simulink model "save"  (R2021a)
settings: Solver=ode4  StartTime=0.0  StopTime=100  FixedStep=0.01  MaxStep=0.01  RelTol=1e-4  EnableMultiTasking=on
undefined symbols (not defined in the file or in its folder): g, k1, k2, k3, m
libraries: pid_lib x1
settings Model: Creator=zlioo  LastModifiedBy=zlioo
settings SolverCC: AlgebraicLoopSolver=TrustRegion
settings DataIOCC: LimitDataPoints=on  SaveOutput=off  SaveTime=off
settings OptimizationCC: ExpressionDepthLimit=2147483647  LifeSpan=1
settings DebuggingCC: UnderspecifiedInitializationDetection=Classic  MergeDetectMultiDrivingBlocksExec=none  FcnCallInpInsideContextMsg=warning  AllowSymbolicDim=off  StateNameClashWarn=warning  SFUnexpectedBacktrackingDiag=warning  SFNoUnconditionalDefaultTransitionDiag=warning  SFExecutionAtInitializationDiag=none  SFMachineParentedDataDiag=warning  ArithmeticOperatorsInVariantConditions=warning
settings SFSimCC: SimUseLocalCustomCode=off  CustomCodeUndefinedFunction=UseInterfaceOnly
settings RTWCC: RTWUseLocalCustomCode=off
settings CodeAppCC: StateflowObjectComments=on
settings GRTTargetCC: TargetLangStandard=C89/C90 (ANSI)  CombineOutputUpdateFcns=off  GRTInterface=on

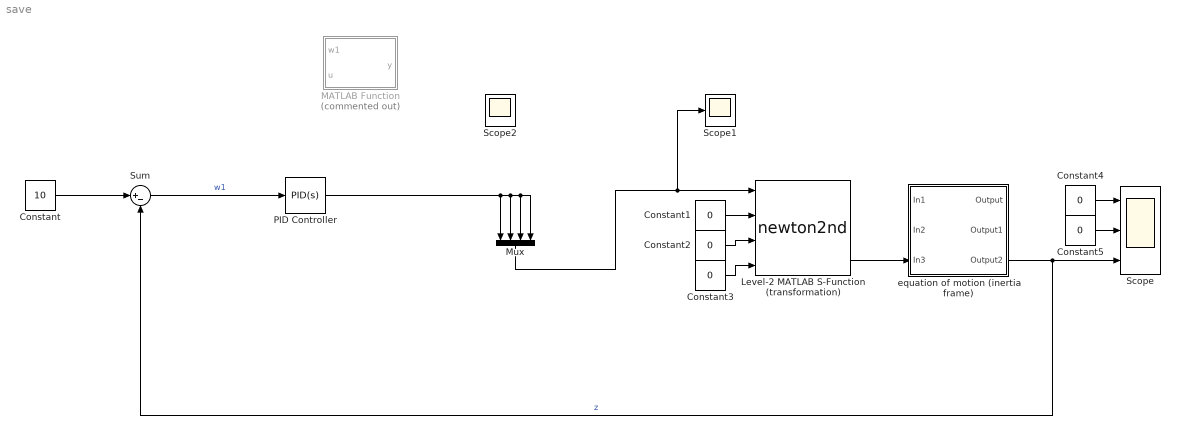
== system save ==
  Constant : Constant  Value=10
  Constant{1..5} (5 alike) : Constant  Value=0
  Level-2 MATLAB S-Function (transformation) : M-S-Function  FunctionName=newton2nd
  MATLAB Function : MATLAB Function  Commented=on  TreatAsAtomicUnit=on
  Mux : Mux
  PID Controller : pid_lib/PID Controller  Controller=PID  Form=Parallel  TimeDomain=Continuous-time  UseExternalTs=off  SampleTime=-1  IntegratorMethod=Forward Euler  FilterMethod=Forward Euler  ControllerParametersSource=internal  P=1.35772493107891  I=0.277456410616241  D=1.63144377299047  UseFilter=on  N=23.8074436453229  TunerSelectOption=Transfer Function Based (PID Tuner App)  InitialConditionSource=internal  InitialConditionForIntegrator=0  InitialConditionForFilter=0  DifferentiatorICPrevScaledInput=0  ExternalReset=none  TrackingMode=off  Kt=1  LimitOutput=off  SatLimitsSource=internal  UpperSaturationLimit=Inf  LowerSaturationLimit=0  LinearizeAsGain=on  AntiWindupMode=none  Kb=1  POutMin=[]  POutMax=[]  IOutMin=[]  IOutMax=[]  DOutMin=[]  DOutMax=[]  NOutMin=[]  NOutMax=[]  SumOutMin=[]  SumOutMax=[]  SaturationOutMin=[]  SaturationOutMax=[]  PParamMin=[]  PParamMax=[]  IParamMin=[]  IParamMax=[]  DParamMin=[]  DParamMax=[]  NParamMin=[]  NParamMax=[]  KbParamMin=[]  KbParamMax=[]  KtParamMin=[]  KtParamMax=[]  KbOutMin=[]  KbOutMax=[]  KtOutMin=[]  KtOutMax=[]  IntegratorOutMin=[]  IntegratorOutMax=[]  FilterOutMin=[]  FilterOutMax=[]  SumI1OutMin=[]  SumI1OutMax=[]  SumI2OutMin=[]  SumI2OutMax=[]  SumI3OutMin=[]  SumI3OutMax=[]  SumI4OutMin=[]  SumI4OutMax=[]  SumDOutMin=[]  SumDOutMax=[]  DifferentiatorOutMin=[]  DifferentiatorOutMax=[]  FilterDiffOutCoefMin=[]  FilterDiffOutCoefMax=[]  ReciprocalOutMin=[]  ReciprocalOutMax=[]  SumDenOutMin=[]  SumDenOutMax=[]  SumNumOutMin=[]  SumNumOutMax=[]  DivideOutMin=[]  DivideOutMax=[]  UdiffTsProdOutMin=[]  UdiffTsProdOutMax=[]  NTsProdOutMin=[]  NTsProdOutMax=[]  UintegralTsProdOutMin=[]  UintegralTsProdOutMax=[]  UngainTsProdOutMin=[]  UngainTsProdOutMax=[]  IntegratorContinuousStateAttributes=''  IntegratorStateMustResolveToSignalObject=off  IntegratorRTWStateStorageClass=Auto  FilterContinuousStateAttributes=''  FilterStateMustResolveToSignalObject=off  FilterRTWStateStorageClass=Auto  ParallelPVariant=InternalParameters  IdealPVariant=Disabled  IVariant=InternalParameters  DVariant=InternalParameters  IntegratorVariant=Continuous  SatVariant=Disabled  AWVariant=Passthrough  PCopyVariant=Disabled  TRVariant=Disabled  FdbkBlocksVariant=Forward  IdealPFdbkVariant=Disabled  SatFdbkVariant=Disabled  DerivativeFilterVariant=ContFilter  NVariant=InternalParameters  NCopyVariant=Disabled  FilterICVariant=InternalICsFilter  IntegratorICVariant=InternalICs  ExternalResetVariant=Disabled  TRSumVariant=Passthrough  SumFdbkVariant=Disabled  SumVariant=Sum_PID  TsampFilterVariant=InternalTs  TsampNgainVariant=Passthrough  TsampIntegralVariant=Passthrough  ExternalSaturationOutDataTypeStr=Inherit: Same as second input
  Scope : Scope  NumInputPorts=3
  Scope1 : Scope
  Scope2 : Scope
  Sum : Sum  Inputs=|+-
  equation of motion (inertia frame) : Subsystem
  wires:
  equation of motion (inertia frame)/3(Output2) -> Scope/3, Sum/2  "z"
  Constant/1 -> Sum/1
  Constant3/1 -> Level-2 MATLAB S-Function (transformation)/4
  Constant2/1 -> Level-2 MATLAB S-Function (transformation)/3
  Constant1/1 -> Level-2 MATLAB S-Function (transformation)/2
  Constant5/1 -> Scope/2
  Constant4/1 -> Scope/1
  Mux/1 -> Scope1/1, Level-2 MATLAB S-Function (transformation)/1
  Level-2 MATLAB S-Function (transformation)/3 -> equation of motion (inertia frame)/3(In3)
  Sum/1 -> PID Controller/1  "w1"
  PID Controller/1 -> Mux/4, Mux/3, Mux/2, Mux/1

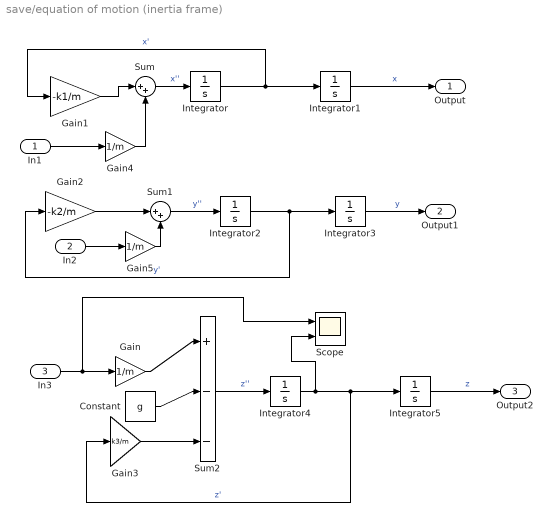
== system save/equation of motion (inertia frame) ==
  In1 : Inport
  In2 : Inport  Port=2
  In3 : Inport  Port=3
  Constant : Constant  Value=g
  Gain : Gain  Gain=1/m
  Gain1 : Gain  Gain=-k1/m
  Gain2 : Gain  Gain=-k2/m
  Gain3 : Gain  Gain=k3/m
  Gain4 : Gain  Gain=1/m
  Gain5 : Gain  Gain=1/m
  Integrator{,1..5} (6 alike) : Integrator
  Scope : Scope  NumInputPorts=2
  Sum : Sum  Inputs=|++
  Sum1 : Sum  Inputs=|++
  Sum2 : Sum  Inputs=|+--
  Output : Outport
  Output1 : Outport  Port=2
  Output2 : Outport  Port=3
  wires:
  Integrator/1 -> Gain1/1, Integrator1/1  "x'"
  Integrator2/1 -> Gain2/1, Integrator3/1  "y'"
  Integrator4/1 -> Scope/2, Integrator5/1, Gain3/1  "z'"
  Sum/1 -> Integrator/1  "x''"
  Gain1/1 -> Sum/1
  Gain2/1 -> Sum1/1
  Sum1/1 -> Integrator2/1  "y''"
  Integrator1/1 -> Output/1  "x"
  Integrator3/1 -> Output1/1  "y"
  Integrator5/1 -> Output2/1  "z"
  In3/1 -> Scope/1, Gain/1
  Gain/1 -> Sum2/1
  Constant/1 -> Sum2/2
  Gain3/1 -> Sum2/3
  Sum2/1 -> Integrator4/1  "z''"
  In1/1 -> Gain4/1
  Gain4/1 -> Sum/2
  In2/1 -> Gain5/1
  Gain5/1 -> Sum1/2

== matlab function save/MATLAB Function ==
  data: w1 input; u input; y output; kf parameter
function y = fcn(w1, u,kf)

y = u;
